simulink model "model_compare"  (R2021b)
settings: Solver=VariableStepAuto  StartTime=0.0  StopTime=1  RelTol=1e-3
libraries: slident x1
settings Model: PauseTimes=0.01  Creator=alexi  LastModifiedBy=alexi

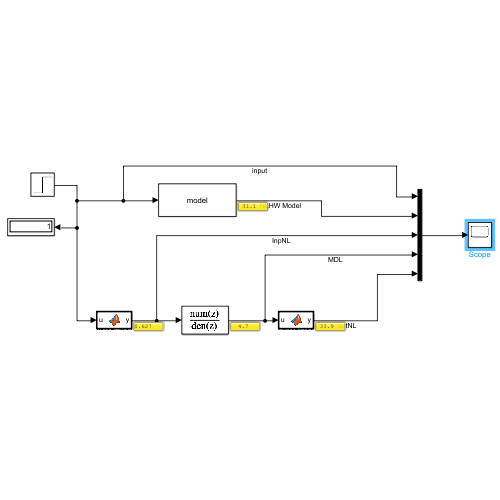
[thumbnail: Simulink's stored preview of the top-level diagram]
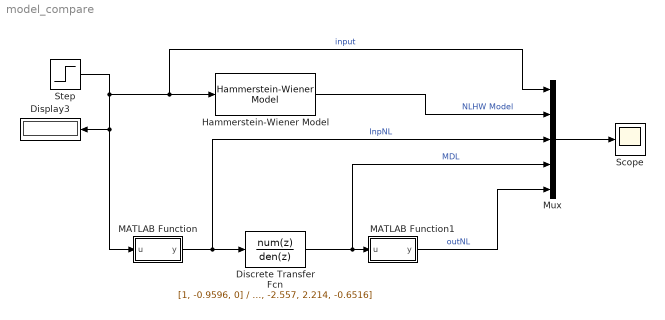
== system model_compare ==
  Discrete Transfer Fcn : DiscreteTransferFcn  Numerator=[1, -0.9596, 0]  Denominator=[1, -2.557, 2.214, -0.6516]  SampleTime=0.01
  Display3 : Display
  Hammerstein-Wiener Model : slident/Models/Hammerstein-Wiener Model  sys=model  IC=Zero  X0i=0
      settings: SourceProductBaseCode=ID
  MATLAB Function : MATLAB Function  TreatAsAtomicUnit=on
  MATLAB Function1 : MATLAB Function  TreatAsAtomicUnit=on
  Mux : Mux  Inputs=5
  Scope : Scope
  Step : Step  Time=0.02  SampleTime=0.01
  wires:
  Step/1 -> Display3/1, MATLAB Function/1(u), Mux/1, Hammerstein-Wiener Model/1  "input"
  MATLAB Function/1(y) -> Discrete Transfer Fcn/1, Mux/3  "InpNL"
  Discrete Transfer Fcn/1 -> Mux/4, MATLAB Function1/1(u)  "MDL"
  MATLAB Function1/1(y) -> Mux/5  "outNL"
  Mux/1 -> Scope/1
  Hammerstein-Wiener Model/1 -> Mux/2  "NLHW Model"

== matlab function model_compare/MATLAB Function ==
  data: u input; y output
function y = inputNonLinearity(u)
    x2 = [-0.4731, 0.2448, 0.419, 0.4531, 0.6003, 0.8796, 1];       
    y2 = [-0.039, 0.0438, 0.1095, 0.1460, 0.2493, 0.5134, 0.627248];
    y = interp1(x2, y2, u);
end

== matlab function model_compare/MATLAB Function1 ==
  data: u input; y output
function y = outputNonLinearity(u)
        x2 = [-4.1721, -2.6285, -0.7644, 0.0366, 0.1922, 1.071, 2.2186, 3.0185, 3.0625, 3.6097, 6.8054, 15];      
        y2 = [-3.1008, -2.8004, 0.2749, -0.0683, 0.0711, 5.0916, 14.0317, 22.6874, 22.5085, 25.7928, 49.701, 111];
        y = interp1(x2, y2, u);
end
